simulink subsystem "Traction_control_old"  (R2022a)
settings: Solver=VariableStepAuto  StartTime=0.0  StopTime=10.0  RelTol=1e-3
settings Model: Creator=jutri  LastModifiedBy=Usuario
settings ModelReferenceCC: EnableRefExpFcnMdlSchedulingChecks=off
settings RTWCC: Description=Generic Real-Time Target  GPUComputeCapability=5.0

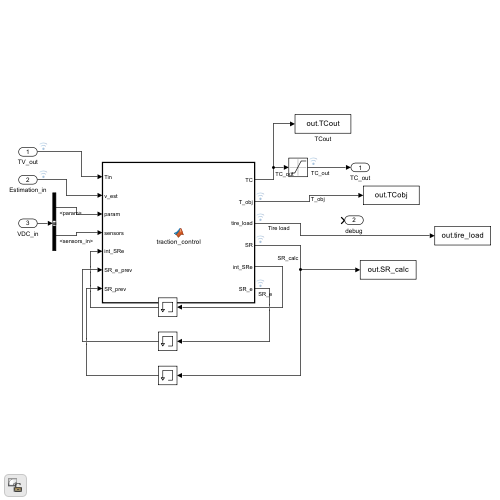
[thumbnail: Simulink's stored preview of the top-level diagram]
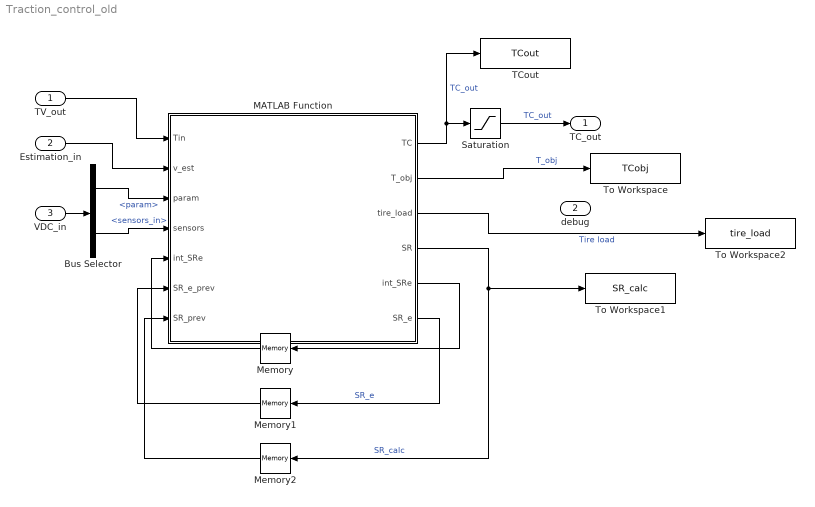
== system Traction_control_old ==
  TV_out : Inport
  Estimation_in : Inport  Port=2
  VDC_in : Inport  Port=3
  Bus Selector : BusSelector  OutputSignals=param,sensors_in
  MATLAB Function : MATLAB Function  TreatAsAtomicUnit=on
  Memory : Memory  InitialCondition=[0;0;0;0]
  Memory1 : Memory  InitialCondition=[0;0;0;0]
  Memory2 : Memory  InitialCondition=[0;0;0;0]
  Saturation : Saturate  UpperLimit=[21; 21; 21; 21]  LowerLimit=[-21; -21; -21; -21]
  TCout : ToWorkspace  VariableName=TCout  SaveFormat=Timeseries  SampleTime=-1
  To Workspace : ToWorkspace  VariableName=TCobj  SaveFormat=Timeseries  SampleTime=-1
  To Workspace1 : ToWorkspace  VariableName=SR_calc  SaveFormat=Timeseries  SampleTime=-1
  To Workspace2 : ToWorkspace  VariableName=tire_load  SaveFormat=Timeseries  SampleTime=-1
  TC_out : Outport
  debug : Outport  Port=2
  wires:
  TV_out/1 -> MATLAB Function/1(Tin)
  Estimation_in/1 -> MATLAB Function/2(v_est)
  MATLAB Function/1(TC) -> Saturation/1, TCout/1  "TC_out"
  VDC_in/1 -> Bus Selector/1
  Bus Selector/1 -> MATLAB Function/3(param)  "<param>"
  Bus Selector/2 -> MATLAB Function/4(sensors)  "<sensors_in>"
  Saturation/1 -> TC_out/1  "TC_out"
  Memory/1 -> MATLAB Function/5("int_SRe ")
  Memory1/1 -> MATLAB Function/6(SR_e_prev)
  MATLAB Function/2(T_obj) -> To Workspace/1  "T_obj"
  MATLAB Function/3(tire_load) -> To Workspace2/1  "Tire load"
  MATLAB Function/4(SR) -> To Workspace1/1, Memory2/1  "SR_calc"
  Memory2/1 -> MATLAB Function/7(SR_prev)
  MATLAB Function/5(int_SRe) -> Memory/1
  MATLAB Function/6(SR_e) -> Memory1/1  "SR_e"

== matlab function Traction_control_old/MATLAB Function ==
  data: Tin input; v_est input; TC output; T_obj output; tire_load output; SR output; int_SRe output; SR_e output; param input; sensors input; int_SRe input; SR_e_prev input; SR_prev input
function [TC, T_obj, tire_load, SR, int_SRe, SR_e] = traction_control(Tin, v_est, param, sensors, int_SRe, SR_e_prev, SR_prev)
% Input:

%  Tin, 
%       Torque Front left TV(1)
%  VDC_in
%  param         - Car's parameters, detailed in vdc-ART25/Parameters.
%       mass, Iz, trackwdidthF, trackwidthR, wheelbase, r_cdg, lf, lr,
%       h_cdg, gear_ratio, rdyn, wheel_inertia, rho, CDA, CLA, g, TimeStep
%  sensors       - Sensor data, stored in struct as follows:
%       IMU
%           r    - Yaw rate [rad/s]
%           ax   - Longitudinal acceleration [m/s^2]
%           ay   - Lateral acceleration [m/s^2]
%       encoder
%           wFL  - Wheelspeed FL [rad/s]
%           wFR  - Wheelspeed FR [rad/s]
%           wRL  - Wheelspeed RL [rad/s]
%           wRR  - Wheelspeed RR [rad/s]
%       ext
%           steering [rad]
%  v_est
%       estimated longitudinal speed

% Output:
%  TC            - Wheel torque after TC
%       Torque Front left
%       Torque Front right
%       Torque Rear left
%       Torque Rear right

if(param.TC_active)

    % Define the gains
    TC_calc = zeros(4,1);
    TC = zeros(4,1);
    SR_e = zeros(4,1);
    
    K  = param.TC_Kp;
    Ki = param.TC_Ti;
    Kd = param.TC_Td;
    Ts = param.TimeStep;
    V0 = param.TC_v0;
    V_gain = param.TC_v_gain;
    
    vx       = v_est(1);
    vy       = v_est(2);
    yaw_rate = v_est(3);
    
    vx_wheel = [vx + 0.5 * yaw_rate * (-param.trackwidthF);
                vx + 0.5 * yaw_rate * ( param.trackwidthF);
                vx + 0.5 * yaw_rate * (-param.trackwidthR);
                vx + 0.5 * yaw_rate * ( param.trackwidthR)];
    
    vy_wheel = [vy + yaw_rate *  param.lf;
                vy + yaw_rate *  param.lf;
                vy + yaw_rate * (-param.lr);
                vy + yaw_rate * (-param.lr)];
    
    cos_steer = cos(sensors.ext.steering);
    sin_steer = sin(sensors.ext.steering);
    
    vx_wheel_tire = [vx_wheel(1) * cos_steer + vy_wheel(1) * sin_steer;
                     vx_wheel(2) * cos_steer + vy_wheel(2) * sin_steer;
                     vx_wheel(3);
                     vx_wheel(4)];
    
    vy_wheel_tire = [-vx_wheel(1) * sin_steer + vy_wheel(1) * cos_steer;
                     -vx_wheel(2) * sin_steer + vy_wheel(2) * cos_steer;
                      vy_wheel(3);
                      vy_wheel(4)];
    
    wr = [sensors.encoder.wFL;
          sensors.encoder.wFR;
          sensors.encoder.wRL;
          sensors.encoder.wRR];
    eps = 0.01;
    
    if vx < 1
        SR = param.rdyn * wr - vx_wheel_tire;
    else
        SR = param.rdyn * wr ./ (vx_wheel_tire + eps) - 1;
    end
    
    SR_t = [0.1; 0.1; 0.1; 0.1];
    
    tire_load = calculate_tire_loads_vdc(sensors.IMU.ax, sensors.IMU.ay, vx, param);
    
    slip_angle = atan2(vy_wheel_tire, vx_wheel_tire);
    
    [~, force_fx, ~, ~] = calculate_tire_forces_vdc(tire_load, slip_angle, SR_t);
    
    inertia_term = (1 + SR_t(1)) * sensors.IMU.ax / param.rdyn * ...
                   param.wheel_inertia / param.gear_ratio;
    
    T_obj = force_fx * param.rdyn / param.gear_ratio + inertia_term;
    
    
    for i = 1:4
        if abs(Tin(i)) < 0.1
            TC_calc(i)   = 0;
            TC(i)        = 0;
            int_SRe(i)   = 0;
            SR_e(i) = 0;
            continue
        end
    
        SR_e(i) = SR_t(i) - abs(SR(i));
        int_SRe(i) = int_SRe(i) + SR_e(i);
    
        pid_calc = K * SR_e(i) ... 
           + Ki * int_SRe(i) ... 
           - Kd * (SR_e(i) - SR_e_prev(i));
    
        TC_calc(i) = T_obj(i) + pid_calc;
        % TC_calc(i) = pid_calc;
    
        TC(i) = min(TC_calc(i), max(Tin(i), -TC_calc(i)));
        if Tin(i) >= 0 && TC_calc(i) < 0
            TC(i) = Tin(i);
        end
    
        if abs(TC_calc(i)) > abs(TC(i))
            int_SRe(i) = 0;
        end
    
    end
    
    if vx < 3
        T_limit = V0 + V_gain * vx;
        if TC(1) > T_limit, TC(1) = T_limit; end
        if TC(2) > T_limit, TC(2) = T_limit; end
    end
    
    for i = 1:4
        if TC(i) > param.torque_limit_positive(i)
            TC(i) = param.torque_limit_positive(i);
        end
        if TC(i) < param.torque_limit_negative(i)
            TC(i) = param.torque_limit_negative(i);
        end
    end
else
    TC = Tin;
    T_obj = zeros(4,1);
    vx = v_est(1);
    tire_load = calculate_tire_loads_vdc(sensors.IMU.ax, sensors.IMU.ay, vx, param);
    SR = zeros(4,1);
    int_SRe = zeros(4,1);
    SR_e = zeros(4,1);
end
